simulink model "cic_example"  (R2014b)
settings: Solver=ode45  StartTime=0.0  StopTime=10.0  RelTol=1e-3
libraries: dspmlti4 x1
settings Model: Creator=Ben  LastModifiedBy=Ben

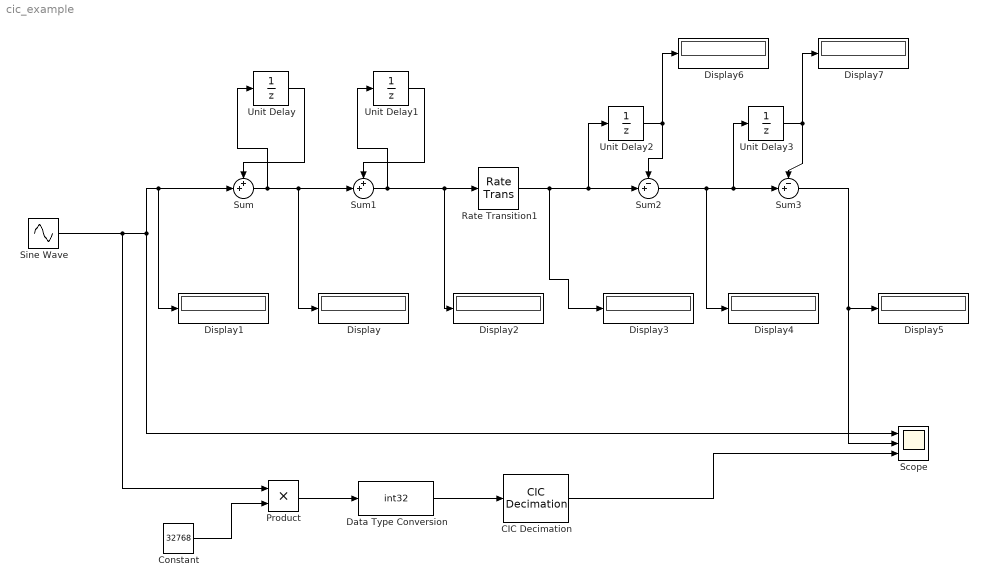
== system cic_example ==
  CIC Decimation : dspmlti4/CIC Decimation  filtFrom=Dialog  filtobj=Hm_decim  ftype=Decimator  R=2  M=1  N=2  filterInternals=Full precision  BPS=[16 16 16 16]  FLPS=0  outputWordLength=32  outputFracLength=0  launchFVT=off  framing=Maintain input frame rate  RateOptions=Allow multirate processing
  Constant : Constant  Value=32768
  Data Type Conversion : DataTypeConversion  OutDataTypeStr=int32
  Display{,1..7} (8 alike) : Display
  Product : Product
  Rate Transition1 : RateTransition  OutPortSampleTime=1/500
  Scope : Scope  NumInputPorts=3
      settings: TimeRange=0.1  YMin=-5~-5~-5  YMax=5~5~5
  Sine Wave : Sin  Frequency=411*pi*2  SampleTime=1/1000
  Sum : Sum  Inputs=++|
  Sum1 : Sum  Inputs=++|
  Sum2 : Sum  Inputs=-+|
  Sum3 : Sum  Inputs=-+|
  Unit Delay{,1..3} (4 alike) : UnitDelay  SampleTime=-1
  wires:
  Sine Wave/1 -> Product/1, Display1/1, Sum/2, Scope/1
  Unit Delay/1 -> Sum/1
  Sum1/1 -> Unit Delay1/1, Display2/1, Rate Transition1/1
  Unit Delay1/1 -> Sum1/1
  Sum/1 -> Display/1, Sum1/2, Unit Delay/1
  Rate Transition1/1 -> Display3/1, Unit Delay2/1, Sum2/2
  Unit Delay2/1 -> Sum2/1, Display6/1
  Sum2/1 -> Display4/1, Unit Delay3/1, Sum3/2
  Unit Delay3/1 -> Sum3/1, Display7/1
  Sum3/1 -> Scope/2, Display5/1
  CIC Decimation/1 -> Scope/3
  Data Type Conversion/1 -> CIC Decimation/1
  Product/1 -> Data Type Conversion/1
  Constant/1 -> Product/2
